simulink model "PC_Quadcopter_Simulation_AE_sslee"  (R2023b)
settings: Solver=ode4  StartTime=0.0  StopTime=40  FixedStep=0.002  MaxStep=0.06  RelTol=1e-3
PreLoadFcn:
  | DoB_parameter
model workspace (MAT data in the model file):
  Sig = Simulink.Signal
  Sig.DataType = 'auto'
  Sig.Dimensions = -1
  Sig.DimensionsMode = 'auto'
  Sig.Complexity = 'auto'
  Sig.SampleTime = -1
  Sig.SamplingMode = 'auto'
values from neighbouring files (symbols this model uses):
  IC = block.DialogPrm(2).Data    [quadcopterDynamicsSFunction.m]
undefined symbols (not defined in the file or in its folder): quadModel
libraries: simulink x14
Description:
  | This is a configurable quadcopter simulation.
  | This Simulink model demonstates position control.
  | 
  | Additional quadcopter modeling and simulation materials available at:
  | github.com/dch33/Quad-Sim
  | 
  | Copyright (C) 2014 D. Hartman, K. Landis, S. Moreno, J. Kim, M. Mehrer
  | 
  | License:
  |     This program is free software: you can redistribute it and/or modify
  |     it under the terms of the GNU LESSER GENERAL PUBLIC LICENSE as published by
  |     the Free Software Foundation, either version 3 of the License, or
  |     (at your option) any later version.
  | 
  |     This program is distributed in the hope that it will be useful,
  |     but WITHOUT ANY WARRANTY; without even the implied warranty of
  |     MERCHANTABILITY or FITNESS FOR A PARTICULAR PURPOSE.  See the
  |     GNU General Public License for more details.
  | 
  |     You should have received a copy of the GNU LESSER GENERAL PUBLIC LICENSE
  |     along with this program.  If not, see <http://www.gnu.org/licenses/>.
settings Model: ModifiedComment=skim -- Tue May 01 16:43:25 2018 -- Version 1.6  Creator=David Hartman  LastModifiedBy=UASG
settings Model: ModifiedHistory=|
  | skim -- Tue May 01 16:43:25 2018 -- Version 1.6
  | 
  | 
  | davidhartman -- Fri Jun 06 22:59:54 2014 -- Version 1.5
settings SolverCC: AlgebraicLoopSolver=TrustRegion
settings DataIOCC: SaveFormat=Array  SignalLogging=off  ReturnWorkspaceOutputs=off
settings OptimizationCC: DefaultParameterBehavior=Inlined  LifeSpan=inf
settings DebuggingCC: SolverPrmCheckMsg=warning  UnconnectedInputMsg=warning  UnconnectedOutputMsg=warning  UnconnectedLineMsg=warning  UniqueDataStoreMsg=warning  StateNameClashWarn=warning  StrictBusMsg=ErrorOnBusTreatedAsVector  SFUnexpectedBacktrackingDiag=warning  SFNoUnconditionalDefaultTransitionDiag=warning  SFExecutionAtInitializationDiag=none  ArithmeticOperatorsInVariantConditions=warning
settings HardwareCC: ProdBitPerPointer=32  ProdBitPerSizeT=32  ProdBitPerPtrDiffT=32  ProdLargestAtomicFloat=None  ProdIntDivRoundTo=Undefined  ProdEndianess=Unspecified  ProdWordSize=32  ProdHWDeviceType=32-bit Generic
settings ModelReferenceCC: EnableRefExpFcnMdlSchedulingChecks=on  PropagateSignalLabelsOutOfModel=off
settings SFSimCC: SimUseLocalCustomCode=off  CustomCodeUndefinedFunction=UseInterfaceOnly
settings RTWCC: RTWUseLocalCustomCode=off  DLArmComputeVersion=19.05
settings CodeAppCC: StateflowObjectComments=on
settings GRTTargetCC: TargetLangStandard=C89/C90 (ANSI)
settings ConfigComp: CovMetricSettings=dw  CovSaveCumulativeToWorkspaceVar=on  CovSaveSingleToWorkspaceVar=on  CovExternalEMLEnable=off

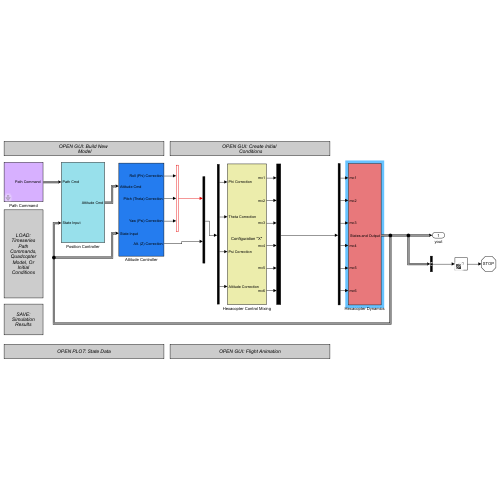
[thumbnail: Simulink's stored preview of the top-level diagram]
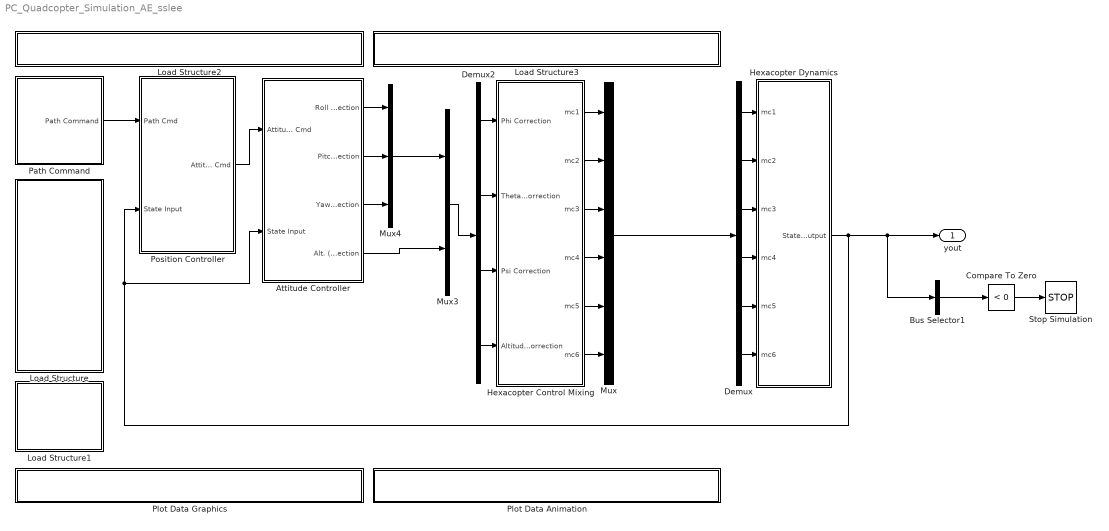
== system PC_Quadcopter_Simulation_AE_sslee ==
  Attitude Controller : Subsystem
  Bus Selector1 : BusSelector  OutputSignals=Z  OutputAsBus=on
  Compare To Zero : simulink/Logic and Bit Operations/Compare To Zero  relop=<  OutDataTypeStr=boolean
  Demux : Demux  Outputs=6
  Demux2 : Demux
  Hexacopter Control Mixing : Subsystem
      mask Display:
      | modelLoaded = evalin('base','exist(''quadModel'',''var'')');
      | if (modelLoaded==1)
      |     if (evalin('base','quadModel.plusConfig'))
      |     fprintf([' \n' ' \n'  'Configuration "+"']);
      |     else if (~evalin('base','quadModel.plusConfig'))
      |         fprintf([' \n' ' \n' 'Configuration "X"']);
      |         end
      |     end
      | else
      |     fprintf([' \n' ' \n'  'Model Not Loaded']);
      | end
  Hexacopter Dynamics : Subsystem
  Load Structure : Subsystem
      settings: OpenFcn=|
      | uiopen('load')
      | if ((exist('IC')==1) && (exist('quadModel')==1) && (exist('path')==1))
      | set_param(bdroot, 'SimulationCommand', 'update')
      | end
      mask Display: fprintf('LOAD:\nTimeseries\nPath\nCommands,\nQuadcopter\nModel, Or\nInitial\nConditions');
  Load Structure1 : Subsystem
      settings: OpenFcn=|
      | if (exist('IC')==1 && exist('quadModel')==1 && exist('yout') && exist('tout'))
      | saveSimResults()
      | else
      | msgbox('No Data To Save!')
      | end
      mask Display: fprintf('SAVE:\nSimulation\nResults');
  Load Structure2 : Subsystem
      settings: OpenFcn=|
      | if exist('GUI_Modeling') == 2,
      | run('GUI_Modeling')
      | 
      | else
      | 
      | msgbox('The desired GUI must be first added to MATLABs path.')
      | 
      | end
      mask Display: fprintf('OPEN GUI: Build New \n Model');
  Load Structure3 : Subsystem
      settings: OpenFcn=|
      | if exist('GUI_IC') == 2,
      | run('GUI_IC')
      | 
      | else
      | 
      | msgbox('The desired GUI must be first added to MATLABs path.')
      | 
      | end
      mask Display: fprintf('OPEN GUI: Create Initial \n Conditions');
  Mux : Mux  Inputs=6
  Mux3 : Mux  Inputs=2
  Mux4 : Mux  Inputs=3
  Path Command : Subsystem  mask{Interpolate=on, OutputAfterFinalValue=Holding final value}
      mask prompts: Interpolate "Interpolate X, Y, Z, and Psi command data?"; OutputAfterFinalValue "Form output after final data value by:"
      mask help:
      | Selecting the Interpolate data checkbox causes position commands to be
      | linearly interpolated. For additional options related to the Timeseries
      | "path" commands, look under the block and click on the Timeseries From
      | Workspace blocks.
      mask TypeOptions Interpolate: X Timeseries From Wkspace/Interpolate | Y Timeseries From Wkspace/Interpolate | Z Timeseries From Wkspace/Interpolate | Psi Timeseries From Wkspace/Interpolate
      mask TypeOptions OutputAfterFinalValue: X Timeseries From Wkspace/OutputAfterFinalValue | Y Timeseries From Wkspace/OutputAfterFinalValue | Z Timeseries From Wkspace/OutputAfterFinalValue | Psi Timeseries From Wkspace/OutputAfterFinalValue
  Plot Data Animation : Subsystem
      settings: OpenFcn=|
      | if exist('QuadAnim4') == 2,
      |     if exist('yout')
      | 	run('QuadAnim4');
      |     else
      |     msgbox('Simulation must be run before data can be plotted.');
      |     end
      | else                                                                          msgbox('The desired GUI must be first added to MATLABs path.')
      | end
      mask Display: fprintf('OPEN GUI: Flight Animation')
  Plot Data Graphics : Subsystem
      settings: OpenFcn=|
      | if exist('yout')
      | yout = evalin('base', 'yout');
      | tout = evalin('base', 'tout');
      | quadPlots(yout, tout)
      | else
      | msgbox('Simulation must be run before data can be plotted.')
      | end
      mask Display: fprintf('OPEN PLOT: State Data')
  Position Controller : Subsystem
  Stop Simulation : Stop
  yout : Outport
  wires:
  Hexacopter Dynamics/1(States and Output) -> Bus Selector1/1, yout/1, Position Controller/2(State Input), Attitude Controller/2(State Input)
  Path Command/1("Path Command ") -> Position Controller/1(Path Cmd)
  Position Controller/1(Attitude Cmd) -> Attitude Controller/1(Attitude Cmd)
  Mux/1 -> Demux/1
  Hexacopter Control Mixing/2(mc2) -> Mux/2
  Hexacopter Control Mixing/3(mc3) -> Mux/3
  Hexacopter Control Mixing/1(mc1) -> Mux/1
  Hexacopter Control Mixing/4(mc4) -> Mux/4
  Demux/3 -> Hexacopter Dynamics/3(mc3)
  Demux/4 -> Hexacopter Dynamics/4(mc4)
  Demux/1 -> Hexacopter Dynamics/1(mc1)
  Demux/2 -> Hexacopter Dynamics/2(mc2)
  Attitude Controller/3(Yaw (Psi) Correction) -> Mux4/3
  Attitude Controller/1(Roll (Phi) Correction) -> Mux4/1
  Attitude Controller/2(Pitch (Theta) Correction) -> Mux4/2
  Demux2/3 -> Hexacopter Control Mixing/3(Psi Correction)
  Demux2/4 -> Hexacopter Control Mixing/4(Altitude Correction)
  Demux2/2 -> Hexacopter Control Mixing/2(Theta Correction)
  Demux2/1 -> Hexacopter Control Mixing/1(Phi Correction)
  Mux4/1 -> Mux3/1
  Attitude Controller/4(Alt. (Z) Correction) -> Mux3/2
  Mux3/1 -> Demux2/1
  Hexacopter Control Mixing/5(mc5) -> Mux/5
  Hexacopter Control Mixing/6(mc6) -> Mux/6
  Demux/5 -> Hexacopter Dynamics/5(mc5)
  Demux/6 -> Hexacopter Dynamics/6(mc6)
  Bus Selector1/1 -> Compare To Zero/1
  Compare To Zero/1 -> Stop Simulation/1

== system PC_Quadcopter_Simulation_AE_sslee/Attitude Controller ==
  Attitude Cmd : Inport
  State Input : Inport  Port=2
  Altitude (Z) Control : Subsystem  mask{Kpz=9, Kiz=6.6, Kdz=9.9, LimitOutput=on, USat=1, LSat=-1, GOffset=(sqrt((quadModel.mass*quadModel.g)/(6*quadModel.ct))-quadModel.b)/quadModel.cr}
      mask prompts: Kpz "Kp"; Kiz "Ki"; Kdz "Kd"; LimitOutput "Integral Saturation?"; USat "Upper saturation limit:"; LSat "Lower saturation limit:"; GOffset "Gravity Feedforward"
      mask help:
      | Adjust PID controller gains through this mask interface, or "look under mask" for more detailed adjustments.
      |
      | Note: Gravity Offset will not appear on block face as a value until simulation is run if it is the result of a formula involving the quadcopter model parameters.
      mask TypeOptions Kpz: Kpz/Gain
      mask TypeOptions Kiz: Kiz/Gain
      mask TypeOptions Kdz: Kdz/Gain
      mask TypeOptions LimitOutput:
      | Integrator
      | Limited/LimitOutput
      mask TypeOptions USat:
      | Integrator
      | Limited/UpperSaturationLimit
      mask TypeOptions LSat:
      | Integrator
      | Limited/LowerSaturationLimit
      mask TypeOptions GOffset: Gravity Offset (Level Flight)/Value
      mask Display:
      | fprintf(['Gravity Offset = ' num2str(GOffset) '\n' ...
      |     'Kp = ' num2str(Kpz) '\n' ...
      |     'Ki = ' num2str(Kiz) '\n' ...
      |     'Kd = ' num2str(Kdz) '\n' ...
      |     'Integral Saturation: ' LimitOutput]);
      | if strcmp(LimitOutput,'on')
      |     fprintf([' \n' ' \n' ' \n' ' \n' ' \n' '\n' ...
      |         'Limits: ' num2str(USat) ' to ' num2str(LSat)]);
      | end
  Bus Selector : BusSelector  OutputSignals=Phi,P,The,Q,Psi,R,Z
  Pitch (Theta) Control : Subsystem  mask{Kpt=2, Kit=1.1, Kdt=1.2, LimitOutput=on, USat=1, LSat=-1}
      mask prompts: Kpt "Kp"; Kit "Ki"; Kdt "Kd"; LimitOutput "Integral Saturation?"; USat "Upper saturation limit:"; LSat "Lower saturation limit:"
      mask help: Adjust PID controller gains through this mask interface, or "look under mask" for more detailed adjustments.
      mask TypeOptions Kpt: Kpt/Gain
      mask TypeOptions Kit: Kit/Gain
      mask TypeOptions Kdt: Kdt/Gain
      mask TypeOptions LimitOutput:
      | Integrator
      | Limited/LimitOutput
      mask TypeOptions USat:
      | Integrator
      | Limited/UpperSaturationLimit
      mask TypeOptions LSat:
      | Integrator
      | Limited/LowerSaturationLimit
      mask Display:
      | fprintf(['Kp = ' num2str(Kpt) '\n' ...
      |     'Ki = ' num2str(Kit) '\n' ...
      |     'Kd = ' num2str(Kdt) '\n' ...
      |     'Integral Saturation: ' LimitOutput]);
      | if strcmp(LimitOutput,'on')
      |     fprintf([' \n' ' \n' ' \n' ' \n' '\n' ...
      |         'Limits: ' num2str(USat) ' to ' num2str(LSat)]);
      | end
  "Roll (Phi) Control " : Subsystem  mask{Kpp=2, Kip=1.1, Kdp=1.2, LimitOutput=on, USat=1, LSat=-1}
      mask prompts: Kpp "Kp"; Kip "Ki"; Kdp "Kd"; LimitOutput "Integral Saturation:"; USat "Upper saturation limit:"; LSat "Lower saturation limit:"
      mask help:
      | Adjust PID controller gains through this mask interface, or "look under mask"
      | for more detailed adjustments.
      mask TypeOptions Kpp: Kpp/Gain
      mask TypeOptions Kip: Kip/Gain
      mask TypeOptions Kdp: Kdp/Gain
      mask TypeOptions LimitOutput:
      | Integrator
      | Limited/LimitOutput
      mask TypeOptions USat:
      | Integrator
      | Limited/UpperSaturationLimit
      mask TypeOptions LSat:
      | Integrator
      | Limited/LowerSaturationLimit
      mask Display:
      | fprintf(['Kp = ' num2str(Kpp) '\n' ...
      |     'Ki = ' num2str(Kip) '\n' ...
      |     'Kd = ' num2str(Kdp) '\n'...
      |     'Integral Saturation: ' LimitOutput]);
      | if strcmp(LimitOutput,'on')
      |     fprintf([' \n' ' \n' ' \n' ' \n' '\n' ...
      |         'Limits: ' num2str(USat) ' to ' num2str(LSat)]);
      | end
  Yaw (Psi) Control : Subsystem  mask{Kps=0.3, Kis=0.15, Kds=0.5, LimitOutput=on, USat=1, LSat=-1}
      mask prompts: Kps "Kp"; Kis "Ki"; Kds "Kd"; LimitOutput "Integral Saturation?"; USat "Upper saturation limit:"; LSat "Lower saturation limit:"
      mask help: Adjust PID controller gains through this mask interface, or "look under mask" for more detailed adjustments.
      mask TypeOptions Kps: Kps/Gain
      mask TypeOptions Kis: Kit/Gain
      mask TypeOptions Kds: Kds/Gain
      mask TypeOptions LimitOutput:
      | Integrator
      | Limited/LimitOutput
      mask TypeOptions USat:
      | Integrator
      | Limited/UpperSaturationLimit
      mask TypeOptions LSat:
      | Integrator
      | Limited/LowerSaturationLimit
      mask Display:
      | fprintf(['Kp = ' num2str(Kps) '\n' ...
      |     'Ki = ' num2str(Kis) '\n' ...
      |     'Kd = ' num2str(Kds) '\n' ...
      |     'Integral Saturation: ' LimitOutput]);
      | if strcmp(LimitOutput,'on')
      |     fprintf([' \n' ' \n' ' \n' ' \n' '\n' ...
      |         'Limits: ' num2str(USat) ' to ' num2str(LSat)]);
      | end
  Roll (Phi) Correction : Outport
  Pitch (Theta) Correction : Outport  Port=2
  Yaw (Psi) Correction : Outport  Port=3
  Alt. (Z) Correction : Outport  Port=4
  wires:
  "Roll (Phi) Control "/1(Phi Correction) -> Roll (Phi) Correction/1
  Bus Selector/1 -> "Roll (Phi) Control "/2(Phi State)  "<Phi>"
  State Input/1 -> Bus Selector/1
  Pitch (Theta) Control/1(Theta Correction) -> Pitch (Theta) Correction/1
  Yaw (Psi) Control/1(Psi Correction) -> Yaw (Psi) Correction/1
  Bus Selector/5 -> Yaw (Psi) Control/2(Psi State)  "<Psi>"
  Altitude (Z) Control/1(Alt. (Z) Correction) -> Alt. (Z) Correction/1
  Bus Selector/7 -> Altitude (Z) Control/2(Z State)  "<Z>"
  Attitude Cmd/1 -> Altitude (Z) Control/1(Desired Z), Yaw (Psi) Control/1(Attitude Command), Pitch (Theta) Control/1(Attitude Command), "Roll (Phi) Control "/1("Attitude Command ")
  Bus Selector/3 -> Pitch (Theta) Control/2(Theta State)  "<The>"
  Bus Selector/2 -> "Roll (Phi) Control "/3(P)  "<P>"
  Bus Selector/4 -> Pitch (Theta) Control/3(P State)  "<Q>"
  Bus Selector/6 -> Yaw (Psi) Control/3(R State)  "<R>"

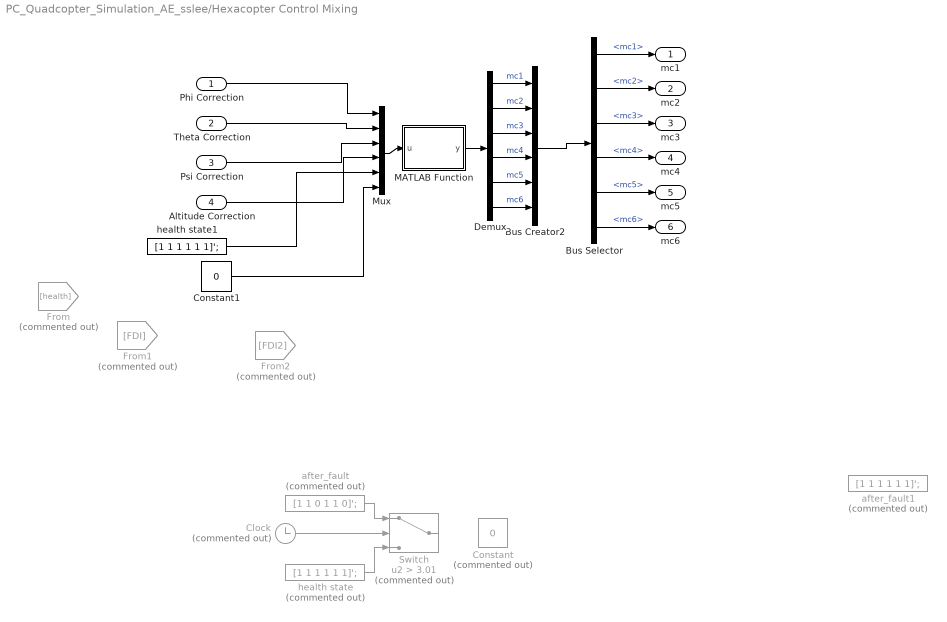
== system PC_Quadcopter_Simulation_AE_sslee/Hexacopter Control Mixing ==
  Phi Correction : Inport
  Theta Correction : Inport  Port=2
  Psi Correction : Inport  Port=3
  Altitude Correction : Inport  Port=4
  Bus Creator2 : BusCreator  Inputs=6
  Bus Selector : BusSelector  OutputSignals=mc1,mc2,mc3,mc4,mc5,mc6
  Clock : Clock  Commented=on
  Constant : Constant  Commented=on  Value=0
  Constant1 : Constant  Value=0
  Demux : Demux  Outputs=6
  From : From  Commented=on  GotoTag=health  TagVisibility=global
  From1 : From  Commented=on  GotoTag=FDI  TagVisibility=global
  From2 : From  Commented=on  GotoTag=FDI2  TagVisibility=global
  MATLAB Function : MATLAB Function  TreatAsAtomicUnit=on
  Mux : Mux  Inputs=6
  Switch : Switch  Commented=on  Criteria=u2 > Threshold  Threshold=3.01  SaturateOnIntegerOverflow=off  InputSameDT=off
  after_fault : Constant  Commented=on  Value=[1 1 0 1 1 0]';
  after_fault1 : Constant  Commented=on  Value=[1 1 1 1 1 1]';
  health state : Constant  Commented=on  Value=[1 1 1 1 1 1]';
  health state1 : Constant  Value=[1 1 1 1 1 1]';
  mc1 : Outport
  mc2 : Outport  Port=2
  mc3 : Outport  Port=3
  mc4 : Outport  Port=4
  mc5 : Outport  Port=5
  mc6 : Outport  Port=6
  wires:
  Phi Correction/1 -> Mux/1
  Theta Correction/1 -> Mux/2
  Psi Correction/1 -> Mux/3
  Altitude Correction/1 -> Mux/4
  Bus Selector/1 -> mc1/1  "<mc1>"
  Bus Selector/2 -> mc2/1  "<mc2>"
  Bus Selector/3 -> mc3/1  "<mc3>"
  Bus Selector/4 -> mc4/1  "<mc4>"
  Bus Selector/5 -> mc5/1  "<mc5>"
  Bus Selector/6 -> mc6/1  "<mc6>"
  Mux/1 -> MATLAB Function/1(u)
  MATLAB Function/1(y) -> Demux/1
  Demux/6 -> Bus Creator2/6  "mc6"
  Demux/3 -> Bus Creator2/3  "mc3"
  Demux/4 -> Bus Creator2/4  "mc4"
  Demux/1 -> Bus Creator2/1  "mc1"
  Demux/5 -> Bus Creator2/5  "mc5"
  Demux/2 -> Bus Creator2/2  "mc2"
  Bus Creator2/1 -> Bus Selector/1
  Constant1/1 -> Mux/6
  health state1/1 -> Mux/5
  health state/1 -> Switch/3
  after_fault/1 -> Switch/1
  Clock/1 -> Switch/2

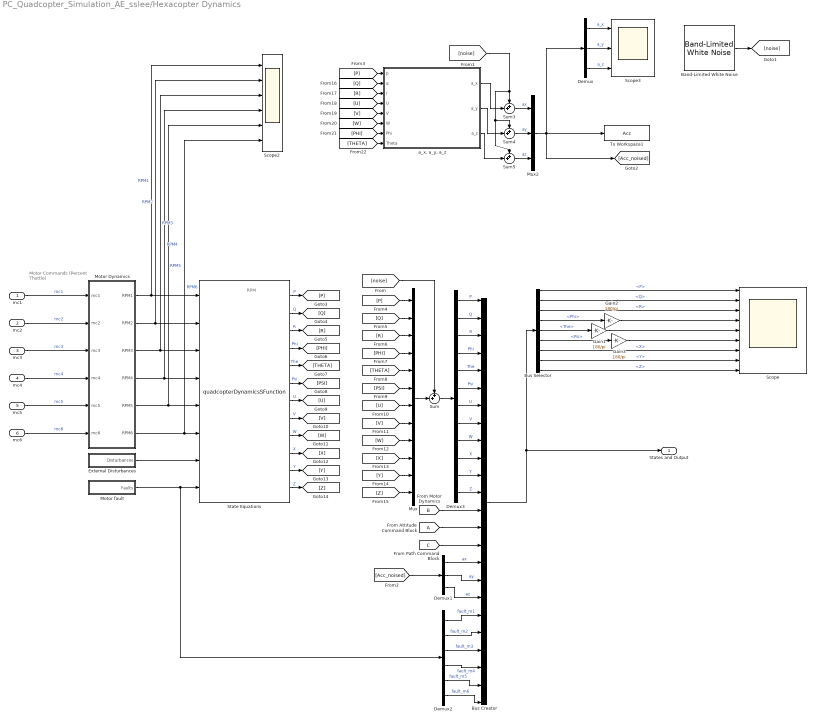
== system PC_Quadcopter_Simulation_AE_sslee/Hexacopter Dynamics ==
  note: RPM
  note: Motor Commands
      | (Percent Thottle)
  mc1 : Inport
  mc2 : Inport  Port=2
  mc3 : Inport  Port=3
  mc4 : Inport  Port=4
  mc5 : Inport  Port=5
  mc6 : Inport  Port=6
  Band-Limited White Noise : simulink/Sources/Band-Limited White Noise  Cov=1e-6  Ts=0.01  seed=[23341]
  Bus Creator : BusCreator  Inputs=24
  Bus Selector : BusSelector  OutputSignals=P,Q,R,Phi,The,Psi,X,Y,Z
  Demux : Demux  Outputs=3
  Demux1 : Demux  Outputs=3
  Demux2 : Demux  Outputs=6
  Demux3 : Demux  Outputs=12
  External Disturbances : Subsystem
  From Attitude Command Block : From  TagVisibility=global
  Gain1 : Gain  Gain=180/pi
  Gain2 : Gain  Gain=180/pi
  Gain3 : Gain  Gain=180/pi
  Motor Dynamics : Subsystem
  Motor fault : Subsystem
  Mux : Mux  Inputs=12
  Mux2 : Mux  Inputs=3
  Scope : Scope  NumInputPorts=9
  Scope2 : Scope  NumInputPorts=6
  Scope3 : Scope  NumInputPorts=3
  State Equations : M-S-Function  FunctionName=quadcopterDynamicsSFunction  Parameters=quadModel, IC
      mask Display:
      | port_label('input', 1, 'RPM1')
      | port_label('input', 2, 'RPM2')
      | port_label('input', 3, 'RPM3')
      | port_label('input', 4, 'RPM4')
      | port_label('input', 5, 'RPM5')
      | port_label('input', 6, 'RPM6')
      | port_label('input', 7, 'Disturbances')
      | port_label('input', 8, 'Faults')
      | port_label('output', 1, 'P')
      | port_label('output', 2, 'Q')
      | port_label('output', 3, 'R')
      | port_label('output', 4, 'Phi')
      | port_label('output', 5, 'The')
      | port_label('output', 6, 'Psi')
      | port_label('output', 7, 'U')
      | port_label('output', 8, 'V')
      | port_label('output', 9, 'W')
      | port_label('output', 10, 'X')
      | port_label('output', 11, 'Y')
      | port_label('output', 12, 'Z')
  Sum{,3..5} (4 alike) : Sum  Inputs=++|
  To Workspace1 : ToWorkspace  VariableName=Acc  SaveFormat=Structure  SampleTime=-1
      settings: Save2DSignal=2-D array (concatenate along first dimension)
  "a_x, a_y, a_z" : Subsystem
  States and Output : Outport
  wires:
  Bus Creator/1 -> Bus Selector/1, States and Output/1
  Motor Dynamics/1(RPM1) -> Scope2/1, State Equations/1  "RPM1"
  Motor Dynamics/2(RPM2) -> Scope2/2, State Equations/2  "RPM2"
  Motor Dynamics/3(RPM3) -> Scope2/3, State Equations/3  "RPM3"
  Motor Dynamics/4(RPM4) -> State Equations/4, Scope2/4  "RPM4"
  mc1/1 -> Motor Dynamics/1(mc1)  "mc1"
  mc4/1 -> Motor Dynamics/4(mc4)  "mc4"
  mc3/1 -> Motor Dynamics/3(mc3)  "mc3"
  mc2/1 -> Motor Dynamics/2(mc2)  "mc2"
  External Disturbances/1("Disturbances ") -> State Equations/7
  From Attitude Command Block/1 -> Bus Creator/14
  [B] -> Bus Creator/13
  [C] -> Bus Creator/15
  mc5/1 -> Motor Dynamics/5(mc5)  "mc5"
  mc6/1 -> Motor Dynamics/6(mc6)  "mc6"
  Motor Dynamics/5(RPM5) -> State Equations/5, Scope2/5  "RPM5"
  Motor Dynamics/6(RPM6) -> State Equations/6, Scope2/6  "RPM6"
  Motor fault/1(Faults) -> Demux2/1, State Equations/8
  Bus Selector/1 -> Scope/1  "<P>"
  Bus Selector/2 -> Scope/2  "<Q>"
  Bus Selector/3 -> Scope/3  "<R>"
  Bus Selector/4 -> Gain2/1  "<Phi>"
  Bus Selector/5 -> Gain1/1  "<The>"
  Bus Selector/6 -> Gain3/1  "<Psi>"
  Bus Selector/7 -> Scope/7  "<X>"
  Bus Selector/8 -> Scope/8  "<Y>"
  Bus Selector/9 -> Scope/9  "<Z>"
  Gain1/1 -> Scope/5
  Gain2/1 -> Scope/4
  Gain3/1 -> Scope/6
  Demux/3 -> Scope3/3  "a_z"
  Demux/2 -> Scope3/2  "a_y"
  Demux/1 -> Scope3/1  "a_x"
  Mux2/1 -> [Acc_noised], To Workspace1/1, Demux/1
  Band-Limited White Noise/1 -> [noise]
  "a_x, a_y, a_z"/1(a_x) -> Sum3/2
  Sum3/1 -> Mux2/1  "ax"
  "a_x, a_y, a_z"/2(a_y) -> Sum4/2
  Sum4/1 -> Mux2/2  "ay"
  "a_x, a_y, a_z"/3(a_z) -> Sum5/2
  Sum5/1 -> Mux2/3  "az"
  [noise] -> Sum5/1, Sum4/1, Sum3/1
  [Acc_noised] -> Demux1/1
  Demux1/1 -> Bus Creator/16  "ax"
  Demux1/2 -> Bus Creator/17  "ay"
  Demux1/3 -> Bus Creator/18  "az"
  Demux2/1 -> Bus Creator/19  "fault_m1"
  Demux2/2 -> Bus Creator/20  "fault_m2"
  Demux2/4 -> Bus Creator/22  "fault_m4"
  Demux2/3 -> Bus Creator/21  "fault_m3"
  Demux2/5 -> Bus Creator/23  "fault_m5"
  Demux2/6 -> Bus Creator/24  "fault_m6"
  State Equations/1 -> [P]  "P"
  State Equations/2 -> [Q]  "Q"
  State Equations/3 -> [R]  "R"
  State Equations/4 -> [PHI]  "Phi"
  State Equations/5 -> [THETA]  "The"
  State Equations/6 -> [PSI]  "Psi"
  State Equations/7 -> [U]  "U"
  State Equations/8 -> [V]  "V"
  State Equations/9 -> [W]  "W"
  State Equations/10 -> [X]  "X"
  State Equations/11 -> [Y]  "Y"
  State Equations/12 -> [Z]  "Z"
  [P] -> "a_x, a_y, a_z"/1(p)
  [Q] -> "a_x, a_y, a_z"/2(q)
  [R] -> "a_x, a_y, a_z"/3(r)
  [U] -> "a_x, a_y, a_z"/4(U)
  [V] -> "a_x, a_y, a_z"/5(V)
  [W] -> "a_x, a_y, a_z"/6(W)
  [THETA] -> "a_x, a_y, a_z"/8(Theta)
  [PHI] -> "a_x, a_y, a_z"/7(Phi)
  [P] -> Mux/1
  [Q] -> Mux/2
  [R] -> Mux/3
  Demux3/1 -> Bus Creator/1  "P"
  Demux3/2 -> Bus Creator/2  "Q"
  Demux3/3 -> Bus Creator/3  "R"
  Mux/1 -> Sum/2
  Sum/1 -> Demux3/1
  [noise] -> Sum/1
  [PHI] -> Mux/4
  [THETA] -> Mux/5
  [PSI] -> Mux/6
  [U] -> Mux/7
  [V] -> Mux/8
  [W] -> Mux/9
  [X] -> Mux/10
  [Y] -> Mux/11
  [Z] -> Mux/12
  Demux3/4 -> Bus Creator/4  "Phi"
  Demux3/5 -> Bus Creator/5  "The"
  Demux3/6 -> Bus Creator/6  "Psi"
  Demux3/7 -> Bus Creator/7  "U"
  Demux3/8 -> Bus Creator/8  "V"
  Demux3/9 -> Bus Creator/9  "W"
  Demux3/10 -> Bus Creator/10  "X"
  Demux3/11 -> Bus Creator/11  "Y"
  Demux3/12 -> Bus Creator/12  "Z"

== system PC_Quadcopter_Simulation_AE_sslee/Load Structure ==

== system PC_Quadcopter_Simulation_AE_sslee/Load Structure1 ==

== system PC_Quadcopter_Simulation_AE_sslee/Load Structure2 ==

== system PC_Quadcopter_Simulation_AE_sslee/Load Structure3 ==

== system PC_Quadcopter_Simulation_AE_sslee/Path Command ==
  Bus Creator : BusCreator  Inputs=4
  Bus Selector : BusSelector  OutputSignals=X_cmd,Y_cmd  OutputAsBus=on
  Psi Timeseries From Wkspace : FromWorkspace  VariableName=path.psi  OutputAfterFinalValue=Holding final value
  X Timeseries From Wkspace : FromWorkspace  VariableName=path.x  OutputAfterFinalValue=Holding final value
  Y Timeseries From Wkspace : FromWorkspace  VariableName=path.y  OutputAfterFinalValue=Holding final value
  Z Timeseries From Wkspace : FromWorkspace  VariableName=path.z  OutputAfterFinalValue=Holding final value
  "Path Command " : Outport
  tag scope: C=global
  wires:
  X Timeseries From Wkspace/1 -> Bus Creator/1  "X_cmd"
  Y Timeseries From Wkspace/1 -> Bus Creator/2  "Y_cmd"
  Z Timeseries From Wkspace/1 -> Bus Creator/3  "Alt_Cmd"
  Psi Timeseries From Wkspace/1 -> Bus Creator/4  "Psi_cmd"
  Bus Creator/1 -> Bus Selector/1, "Path Command "/1  "Path_Cmd"
  Bus Selector/1 -> [C]  "XY_Cmd"

== system PC_Quadcopter_Simulation_AE_sslee/Plot Data Animation ==

== system PC_Quadcopter_Simulation_AE_sslee/Plot Data Graphics ==

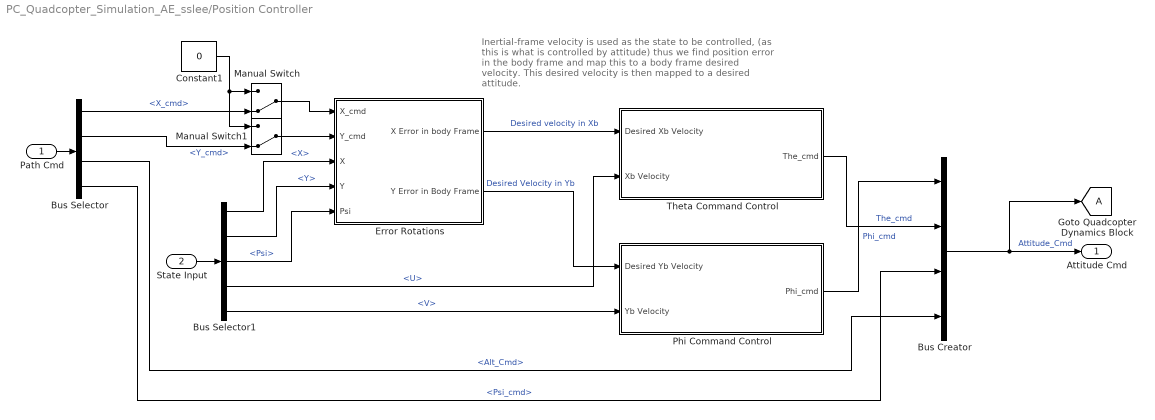
== system PC_Quadcopter_Simulation_AE_sslee/Position Controller ==
  note: Inertial-frame velocity is used as the state to be controlled,
      | (as this is what is controlled by attitude)
      | thus we find position error in the body frame
      | and map this to a body frame desired velocity. This desired
      | velocity is then mapped to a desired attitude.
  Path Cmd : Inport
  State Input : Inport  Port=2
  Bus Creator : BusCreator  Inputs=4
  Bus Selector : BusSelector  OutputSignals=X_cmd,Y_cmd,Alt_Cmd,Psi_cmd
  Bus Selector1 : BusSelector  OutputSignals=X,Y,Psi,U,V
  Constant1 : Constant  Value=0
  Error Rotations : Subsystem
  Goto Quadcopter Dynamics Block : Goto  TagVisibility=global
  Manual Switch : ManualSwitch  CurrentSetting=0
  Manual Switch1 : ManualSwitch  CurrentSetting=0
  Phi Command Control : Subsystem  mask{Kp=0.32, Kd=0.1, ASat=20*pi/180}
      mask prompts: Kp "Proportional Gain"; Kd "Derivative Gain"; ASat "Attitude Limit (+/- radians):"
      mask TypeOptions Kp: Kpp/Gain
      mask TypeOptions Kd: Kdp/Gain
      mask TypeOptions ASat: Attitude Limits_Phi/UpperLimit
      mask Display:
      | fprintf(['Kp = ' num2str(Kp) '\n' ...
      |     'Kd = ' num2str(Kd) '\n' ...
      |     'Attitude Limit (+/-): ' num2str(ASat*180/pi) '°']);
  Theta Command Control : Subsystem  mask{Kp=0.32, Kd=0.1, ASat=20*pi/180}
      mask prompts: Kp "Proportional Gain:"; Kd "Derivative Gain"; ASat "Attitude Limit (+/- radians):"
      mask TypeOptions Kp: Kpt/Gain
      mask TypeOptions Kd: Kdt/Gain
      mask TypeOptions ASat: Attitude Limits_Theta/UpperLimit
      mask Display:
      | fprintf(['Kp = ' num2str(Kp) '\n' ...
      |     'Kd = ' num2str(Kd) '\n' ...
      |     'Attitude Limit (+/-): ' num2str(ASat*180/pi) '°']);
  Attitude Cmd : Outport
  wires:
  Bus Selector1/5 -> Phi Command Control/2(Yb Velocity)  "<V>"
  State Input/1 -> Bus Selector1/1
  Bus Selector/4 -> Bus Creator/3  "<Psi_cmd>"
  Path Cmd/1 -> Bus Selector/1
  Bus Selector/3 -> Bus Creator/4  "<Alt_Cmd>"
  Bus Creator/1 -> Attitude Cmd/1, Goto Quadcopter Dynamics Block/1  "Attitude_Cmd"
  Bus Selector/1 -> Manual Switch/2  "<X_cmd>"
  Bus Selector1/1 -> Error Rotations/3(X)  "<X>"
  Bus Selector1/2 -> Error Rotations/4(Y)  "<Y>"
  Bus Selector1/3 -> Error Rotations/5(Psi)  "<Psi>"
  Error Rotations/1(X Error in body Frame) -> Theta Command Control/1(Desired Xb Velocity)  "Desired velocity in Xb"
  Bus Selector1/4 -> Theta Command Control/2(Xb Velocity)  "<U>"
  Theta Command Control/1(The_cmd) -> Bus Creator/2  "The_cmd"
  Error Rotations/2(Y Error in Body Frame) -> Phi Command Control/1(Desired Yb Velocity)  "Desired Velocity in Yb"
  Phi Command Control/1(Phi_cmd) -> Bus Creator/1  "Phi_cmd"
  Constant1/1 -> Manual Switch1/1, Manual Switch/1
  Manual Switch/1 -> Error Rotations/1(X_cmd)
  Bus Selector/2 -> Manual Switch1/2  "<Y_cmd>"
  Manual Switch1/1 -> Error Rotations/2(Y_cmd)

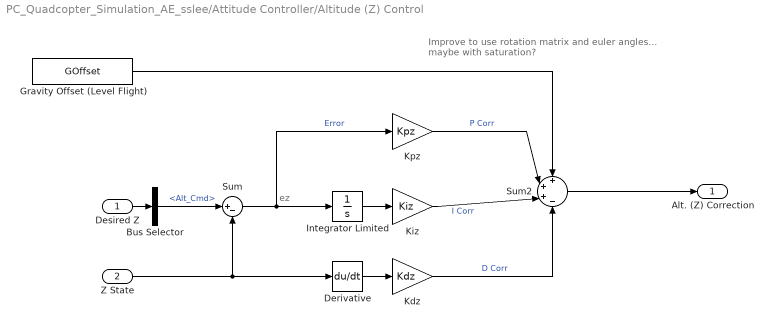
== system PC_Quadcopter_Simulation_AE_sslee/Attitude Controller/Altitude (Z) Control ==
  note: Improve to use rotation matrix and euler angles...
      | maybe with saturation?
  note: ez
  Desired Z : Inport
  Z State : Inport  Port=2
  Bus Selector : BusSelector  OutputSignals=Alt_Cmd
  Derivative : Derivative
  Gravity Offset (Level Flight) : Constant  Value=GOffset
  Integrator Limited : Integrator  LimitOutput=on  UpperSaturationLimit=USat  LowerSaturationLimit=LSat
  Kdz : Gain  Gain=Kdz
  Kiz : Gain  Gain=Kiz
  Kpz : Gain  Gain=Kpz
  Sum : Sum  Inputs=|+-
  Sum2 : Sum  Inputs=+++-
  Alt. (Z) Correction : Outport
  wires:
  Gravity Offset (Level Flight)/1 -> Sum2/1
  Desired Z/1 -> Bus Selector/1
  Z State/1 -> Derivative/1, Sum/2
  Sum2/1 -> Alt. (Z) Correction/1
  Kpz/1 -> Sum2/2  "P Corr"
  Sum/1 -> Integrator Limited/1, Kpz/1  "Error"
  Kiz/1 -> Sum2/3  "I Corr"
  Kdz/1 -> Sum2/4  "D Corr"
  Integrator Limited/1 -> Kiz/1
  Bus Selector/1 -> Sum/1  "<Alt_Cmd>"
  Derivative/1 -> Kdz/1

== system PC_Quadcopter_Simulation_AE_sslee/Attitude Controller/Pitch (Theta) Control ==
  Attitude Command : Inport
  Theta State : Inport  Port=2
  P State : Inport  Port=3
  Bus Selector : BusSelector  OutputSignals=The_cmd
  Integrator Limited : Integrator  LimitOutput=on  UpperSaturationLimit=USat  LowerSaturationLimit=LSat
  Kdt : Gain  Gain=Kdt
  Kit : Gain  Gain=Kit
  Kpt : Gain  Gain=Kpt
  Sum : Sum  Inputs=|+-
  Sum1 : Sum  Inputs=++-
  Theta Correction : Outport
  wires:
  Sum/1 -> Integrator Limited/1, Kpt/1  "Error"
  Attitude Command/1 -> Bus Selector/1
  Theta State/1 -> Sum/2
  Sum1/1 -> Theta Correction/1
  Kpt/1 -> Sum1/1  "P Corr"
  Kdt/1 -> Sum1/3  "D Corr"
  Kit/1 -> Sum1/2  "I Corr"
  Integrator Limited/1 -> Kit/1
  Bus Selector/1 -> Sum/1  "<The_cmd>"
  P State/1 -> Kdt/1

== system PC_Quadcopter_Simulation_AE_sslee/Attitude Controller/Roll (Phi) Control  ==
  "Attitude Command " : Inport
  Phi State : Inport  Port=2
  P : Inport  Port=3
  Bus Selector : BusSelector  OutputSignals=Phi_cmd
  Integrator Limited : Integrator  LimitOutput=on  UpperSaturationLimit=USat  LowerSaturationLimit=LSat
  Kdp : Gain  Gain=Kdp
  Kip : Gain  Gain=Kip
  Kpp : Gain  Gain=Kpp
  Sum : Sum  Inputs=|+-
  Sum1 : Sum  Inputs=++-
  Phi Correction : Outport
  wires:
  Sum/1 -> Integrator Limited/1, Kpp/1  "Error"
  Phi State/1 -> Sum/2
  Sum1/1 -> Phi Correction/1
  Kpp/1 -> Sum1/1  "P Corr"
  Kdp/1 -> Sum1/3  "D Corr"
  Kip/1 -> Sum1/2  "I Corr"
  Integrator Limited/1 -> Kip/1
  "Attitude Command "/1 -> Bus Selector/1
  Bus Selector/1 -> Sum/1  "<Phi_cmd>"
  P/1 -> Kdp/1

== system PC_Quadcopter_Simulation_AE_sslee/Attitude Controller/Yaw (Psi) Control ==
  Attitude Command : Inport
  Psi State : Inport  Port=2
  R State : Inport  Port=3
  Bus Selector : BusSelector  OutputSignals=Psi_cmd
  Integrator Limited : Integrator  LimitOutput=on  UpperSaturationLimit=USat  LowerSaturationLimit=LSat
  Kds : Gain  Gain=Kds
  Kit : Gain  Gain=Kis
  Kps : Gain  Gain=Kps
  Sum : Sum  Inputs=|+-
  Sum1 : Sum  Inputs=++-
  Psi Correction : Outport
  wires:
  Sum/1 -> Integrator Limited/1, Kps/1  "Error"
  Attitude Command/1 -> Bus Selector/1
  Sum1/1 -> Psi Correction/1
  Psi State/1 -> Sum/2
  Kps/1 -> Sum1/1  "P Corr"
  Kds/1 -> Sum1/3  "D Corr"
  Kit/1 -> Sum1/2  "I Corr"
  Integrator Limited/1 -> Kit/1
  Bus Selector/1 -> Sum/1  "<Psi_cmd>"
  R State/1 -> Kds/1

== system PC_Quadcopter_Simulation_AE_sslee/Hexacopter Dynamics/External Disturbances ==
  note: Note: Torques are in units of N*m, Forces in N
      | Torques are applied to the BODY coordinate system.
      | Forces are applied from the WORLD coordinate system!
      | This can be changed by adjusting the equations within the S-function.
  Bus Creator : BusCreator  Inputs=6
  Bus to Vector : BusToVector
  Constant{1..2,5..6} (4 alike) : Constant  Value=0
  Manual Switch : ManualSwitch
  Manual Switch1 : ManualSwitch
  Step : Step  Time=5  After=0.1  SampleTime=0
  Step2 : Step  Time=10  After=3  SampleTime=0
  "Disturbances " : Outport
  wires:
  Bus to Vector/1 -> "Disturbances "/1
  Bus Creator/1 -> Bus to Vector/1
  Constant6/1 -> Manual Switch1/1, Bus Creator/1  "Tau_bx-axis"
  Constant2/1 -> Bus Creator/3  "Tau_bz-axis"
  Constant1/1 -> Manual Switch/1, Bus Creator/4  "Force_x-axis"
  Constant5/1 -> Bus Creator/6  "Force_z-axis"
  Manual Switch/1 -> Bus Creator/5
  Step2/1 -> Manual Switch/2  "Force_y-axis"
  Manual Switch1/1 -> Bus Creator/2
  Step/1 -> Manual Switch1/2  "Tau_by-axis"

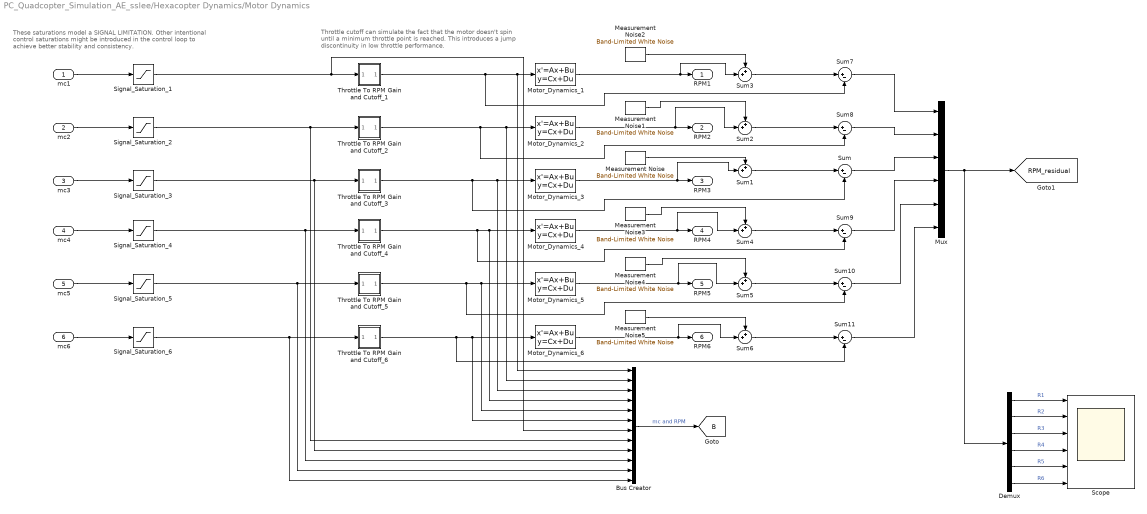
== system PC_Quadcopter_Simulation_AE_sslee/Hexacopter Dynamics/Motor Dynamics ==
  note: Throttle cutoff can simulate the fact that the motor doesn't
      | spin until a minimum throttle point is reached. This introduces
      | a jump discontinuity in low throttle performance.
  note: These saturations model a SIGNAL LIMITATION.
      | Other intentional control saturations might be introduced in the
      | control loop to achieve better stability and consistency.
  mc1 : Inport
  mc2 : Inport  Port=2
  mc3 : Inport  Port=3
  mc4 : Inport  Port=4
  mc5 : Inport  Port=5
  mc6 : Inport  Port=6
  Bus Creator : BusCreator  Inputs=12
  Demux : Demux  Outputs=6
  Measurement Noise{,1..5} (6 alike) : simulink/Sources/Band-Limited White Noise  Cov=10^2  Ts=0.02  seed=[23342]
  Motor_Dynamics_1 : StateSpace  A=-1/quadModel.T  C=1/quadModel.T  D=0  InitialCondition=IC.w1*quadModel.T
  Motor_Dynamics_2 : StateSpace  A=-1/quadModel.T  C=1/quadModel.T  D=0  InitialCondition=IC.w2*quadModel.T
  Motor_Dynamics_3 : StateSpace  A=-1/quadModel.T  C=1/quadModel.T  D=0  InitialCondition=IC.w3*quadModel.T
  Motor_Dynamics_4 : StateSpace  A=-1/quadModel.T  C=1/quadModel.T  D=0  InitialCondition=IC.w4*quadModel.T
  Motor_Dynamics_5 : StateSpace  A=-1/quadModel.T  C=1/quadModel.T  D=0  InitialCondition=IC.w4*quadModel.T
  Motor_Dynamics_6 : StateSpace  A=-1/quadModel.T  C=1/quadModel.T  D=0  InitialCondition=IC.w4*quadModel.T
  Mux : Mux  Inputs=6
  Scope : Scope  NumInputPorts=6
  Signal_Saturation_{1..6} (6 alike) : Saturate  UpperLimit=100  LowerLimit=0
  Sum{,7..11} (6 alike) : Sum  Inputs=|+-
  Sum{1..6} (6 alike) : Sum  Inputs=++|
  Throttle To RPM Gain and Cutoff_1 : Subsystem
  Throttle To RPM Gain and Cutoff_2 : Subsystem
  Throttle To RPM Gain and Cutoff_3 : Subsystem
  Throttle To RPM Gain and Cutoff_4 : Subsystem
  Throttle To RPM Gain and Cutoff_5 : Subsystem
  Throttle To RPM Gain and Cutoff_6 : Subsystem
  RPM1 : Outport
  RPM2 : Outport  Port=2
  RPM3 : Outport  Port=3
  RPM4 : Outport  Port=4
  RPM5 : Outport  Port=5
  RPM6 : Outport  Port=6
  tag scope: B=global, RPM_residual=global
  wires:
  mc1/1 -> Signal_Saturation_1/1
  mc4/1 -> Signal_Saturation_4/1
  mc2/1 -> Signal_Saturation_2/1
  mc3/1 -> Signal_Saturation_3/1
  Signal_Saturation_1/1 -> Bus Creator/7, Throttle To RPM Gain and Cutoff_1/1(In5)
  Signal_Saturation_2/1 -> Throttle To RPM Gain and Cutoff_2/1(In5), Bus Creator/8
  Signal_Saturation_3/1 -> Bus Creator/9, Throttle To RPM Gain and Cutoff_3/1(In5)
  Signal_Saturation_4/1 -> Bus Creator/10, Throttle To RPM Gain and Cutoff_4/1(In5)
  Throttle To RPM Gain and Cutoff_1/1(Out5) -> Sum7/2, Bus Creator/1, Motor_Dynamics_1/1
  Throttle To RPM Gain and Cutoff_2/1(Out5) -> Sum8/2, Motor_Dynamics_2/1, Bus Creator/2
  Throttle To RPM Gain and Cutoff_3/1(Out5) -> Sum/2, Motor_Dynamics_3/1, Bus Creator/3
  Throttle To RPM Gain and Cutoff_4/1(Out5) -> Sum9/2, Motor_Dynamics_4/1, Bus Creator/4
  Motor_Dynamics_1/1 -> Sum3/2, RPM1/1
  Motor_Dynamics_2/1 -> Sum2/2, RPM2/1
  Motor_Dynamics_3/1 -> Sum1/2, RPM3/1
  Motor_Dynamics_4/1 -> Sum4/2, RPM4/1
  Bus Creator/1 -> [B]  "mc and RPM"
  Motor_Dynamics_5/1 -> Sum5/2, RPM5/1
  mc5/1 -> Signal_Saturation_5/1
  Signal_Saturation_5/1 -> Bus Creator/11, Throttle To RPM Gain and Cutoff_5/1(In5)
  Throttle To RPM Gain and Cutoff_5/1(Out5) -> Sum10/2, Motor_Dynamics_5/1, Bus Creator/5
  Motor_Dynamics_6/1 -> Sum6/2, RPM6/1
  mc6/1 -> Signal_Saturation_6/1
  Signal_Saturation_6/1 -> Bus Creator/12, Throttle To RPM Gain and Cutoff_6/1(In5)
  Throttle To RPM Gain and Cutoff_6/1(Out5) -> Sum11/2, Motor_Dynamics_6/1, Bus Creator/6
  Mux/1 -> Demux/1, [RPM_residual]
  Measurement Noise/1 -> Sum1/1
  Sum1/1 -> Sum/1
  Measurement Noise5/1 -> Sum6/1
  Measurement Noise4/1 -> Sum5/1
  Measurement Noise3/1 -> Sum4/1
  Measurement Noise1/1 -> Sum2/1
  Measurement Noise2/1 -> Sum3/1
  Sum2/1 -> Sum8/1
  Sum3/1 -> Sum7/1
  Sum4/1 -> Sum9/1
  Sum5/1 -> Sum10/1
  Sum6/1 -> Sum11/1
  Sum7/1 -> Mux/1
  Sum8/1 -> Mux/2
  Sum/1 -> Mux/3
  Sum9/1 -> Mux/4
  Sum10/1 -> Mux/5
  Sum11/1 -> Mux/6
  Demux/6 -> Scope/6  "R6"
  Demux/5 -> Scope/5  "R5"
  Demux/4 -> Scope/4  "R4"
  Demux/3 -> Scope/3  "R3"
  Demux/2 -> Scope/2  "R2"
  Demux/1 -> Scope/1  "R1"

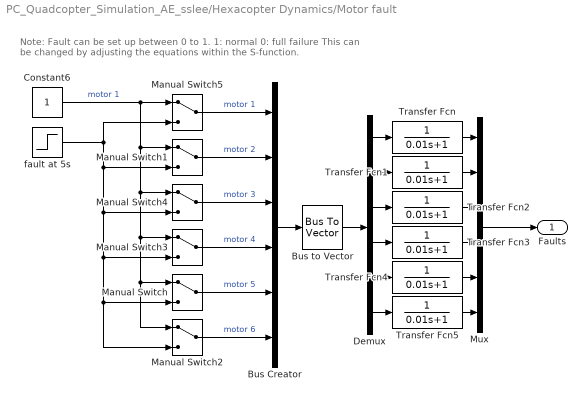
== system PC_Quadcopter_Simulation_AE_sslee/Hexacopter Dynamics/Motor fault ==
  note: Note: Fault can be set up between 0 to 1.
      | 1: normal
      | 0: full failure
      | This can be changed by adjusting the equations within the S-function.
  Bus Creator : BusCreator  Inputs=6
  Bus to Vector : BusToVector
  Constant6 : Constant
  Demux : Demux  Outputs=6
  Manual Switch{,1..5} (6 alike) : ManualSwitch
  Mux : Mux  Inputs=6
  Transfer Fcn{,1..5} (6 alike) : TransferFcn  Numerator=1  Denominator=[0.01 1]
  fault at 5s : Step  Time=30  Before=1  After=0  SampleTime=0
  Faults : Outport
  wires:
  Manual Switch1/1 -> Bus Creator/2  "motor 2"
  Manual Switch/1 -> Bus Creator/5  "motor 5"
  Bus Creator/1 -> Bus to Vector/1
  Manual Switch2/1 -> Bus Creator/6  "motor 6"
  Manual Switch3/1 -> Bus Creator/4  "motor 4"
  Demux/1 -> Transfer Fcn/1
  Demux/2 -> Transfer Fcn1/1
  Demux/3 -> Transfer Fcn2/1
  Demux/6 -> Transfer Fcn5/1
  Demux/5 -> Transfer Fcn4/1
  Demux/4 -> Transfer Fcn3/1
  Transfer Fcn/1 -> Mux/1
  Transfer Fcn1/1 -> Mux/2
  Transfer Fcn2/1 -> Mux/3
  Transfer Fcn4/1 -> Mux/5
  Transfer Fcn5/1 -> Mux/6
  Transfer Fcn3/1 -> Mux/4
  Manual Switch4/1 -> Bus Creator/3  "motor 3"
  Constant6/1 -> Manual Switch5/1, Manual Switch2/1, Manual Switch/1, Manual Switch3/1, Manual Switch4/1, Manual Switch1/1  "motor 1"
  Manual Switch5/1 -> Bus Creator/1  "motor 1"
  fault at 5s/1 -> Manual Switch2/2, Manual Switch/2, Manual Switch3/2, Manual Switch4/2, Manual Switch1/2, Manual Switch5/2
  Bus to Vector/1 -> Demux/1
  Mux/1 -> Faults/1

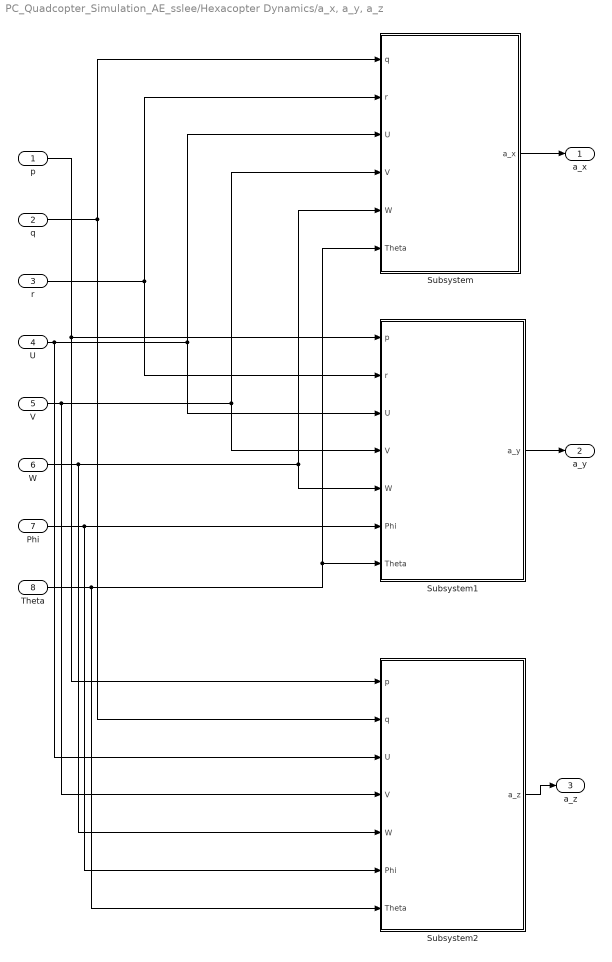
== system PC_Quadcopter_Simulation_AE_sslee/Hexacopter Dynamics/a_x, a_y, a_z ==
  p : Inport
  q : Inport  Port=2
  r : Inport  Port=3
  U : Inport  Port=4
  V : Inport  Port=5
  W : Inport  Port=6
  Phi : Inport  Port=7
  Theta : Inport  Port=8
  Subsystem : Subsystem
  Subsystem1 : Subsystem
  Subsystem2 : Subsystem
  a_x : Outport
  a_y : Outport  Port=2
  a_z : Outport  Port=3
  wires:
  Subsystem/1(a_x) -> a_x/1
  Subsystem1/1(a_y) -> a_y/1
  Subsystem2/1(a_z) -> a_z/1
  q/1 -> Subsystem2/2(q), Subsystem/1(q)
  r/1 -> Subsystem/2(r), Subsystem1/2(r)
  U/1 -> Subsystem2/3(U), Subsystem1/3(U), Subsystem/3(U)
  V/1 -> Subsystem2/4(V), Subsystem/4(V), Subsystem1/4(V)
  W/1 -> Subsystem2/5(W), Subsystem/5(W), Subsystem1/5(W)
  Theta/1 -> Subsystem2/7(Theta), Subsystem1/7(Theta), Subsystem/6(Theta)
  p/1 -> Subsystem2/1(p), Subsystem1/1(p)
  Phi/1 -> Subsystem2/6(Phi), Subsystem1/6(Phi)

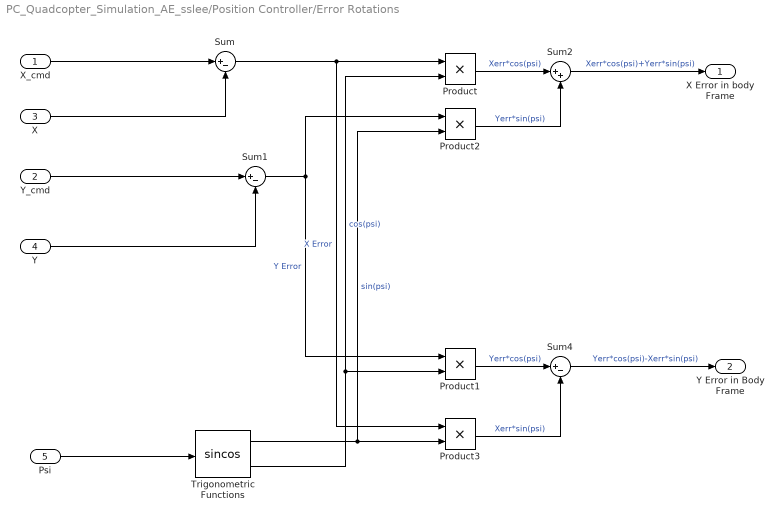
== system PC_Quadcopter_Simulation_AE_sslee/Position Controller/Error Rotations ==
  X_cmd : Inport
  Y_cmd : Inport  Port=2
  X : Inport  Port=3
  Y : Inport  Port=4
  Psi : Inport  Port=5
  Product{,1..3} (4 alike) : Product
  Sum : Sum  Inputs=|+-
  Sum1 : Sum  Inputs=|+-
  Sum2 : Sum  Inputs=|++
  Sum4 : Sum  Inputs=|+-
  Trigonometric Functions : Trigonometry  Operator=sincos
  X Error in body Frame : Outport
  Y Error in Body Frame : Outport  Port=2
  wires:
  Sum4/1 -> Y Error in Body Frame/1  "Yerr*cos(psi)-Xerr*sin(psi)"
  Product3/1 -> Sum4/2  "Xerr*sin(psi)"
  Sum1/1 -> Product2/1, Product1/1  "Y Error"
  Trigonometric Functions/1 -> Product2/2, Product3/2  "sin(psi)"
  Sum2/1 -> X Error in body Frame/1  "Xerr*cos(psi)+Yerr*sin(psi)"
  Y_cmd/1 -> Sum1/1
  X_cmd/1 -> Sum/1
  X/1 -> Sum/2
  Y/1 -> Sum1/2
  Sum/1 -> Product3/1, Product/1  "X Error"
  Trigonometric Functions/2 -> Product/2, Product1/2  "cos(psi)"
  Product/1 -> Sum2/1  "Xerr*cos(psi)"
  Product2/1 -> Sum2/2  "Yerr*sin(psi)"
  Product1/1 -> Sum4/1  "Yerr*cos(psi)"
  Psi/1 -> Trigonometric Functions/1

== system PC_Quadcopter_Simulation_AE_sslee/Position Controller/Phi Command Control ==
  note: -1 Gain is required because a "negative"
      | angle of Phi induces a positive velocity
      | in the body frame y direction!
  Desired Yb Velocity : Inport
  Yb Velocity : Inport  Port=2
  Attitude Limits_Phi : Saturate  UpperLimit=ASat  LowerLimit=-ASat
  Gain : Gain  Gain=-1
  Kdp : Gain  Gain=Kd
  Kpp : Gain  Gain=Kp
  Sum3 : Sum  Inputs=|+-
  Sum6 : Sum  Inputs=|+-
  V Derivative : Derivative
  Phi_cmd : Outport
  wires:
  V Derivative/1 -> Kdp/1
  Attitude Limits_Phi/1 -> Phi_cmd/1  "Phi_cmd"
  Sum6/1 -> Gain/1
  Kpp/1 -> Sum6/1
  Sum3/1 -> Kpp/1  "Velocity Error"
  Yb Velocity/1 -> V Derivative/1, Sum3/2
  Desired Yb Velocity/1 -> Sum3/1
  Gain/1 -> Attitude Limits_Phi/1
  Kdp/1 -> Sum6/2

== system PC_Quadcopter_Simulation_AE_sslee/Position Controller/Theta Command Control ==
  Desired Xb Velocity : Inport
  Xb Velocity : Inport  Port=2
  Attitude Limits_Theta : Saturate  UpperLimit=ASat  LowerLimit=-ASat
  Kdt : Gain  Gain=Kd
  Kpt : Gain  Gain=Kp
  Sum3 : Sum  Inputs=|+-
  Sum6 : Sum  Inputs=|+-
  U Derivative : Derivative
  The_cmd : Outport
  wires:
  Kdt/1 -> Sum6/2
  U Derivative/1 -> Kdt/1
  Attitude Limits_Theta/1 -> The_cmd/1  "The_cmd"
  Sum6/1 -> Attitude Limits_Theta/1
  Kpt/1 -> Sum6/1
  Sum3/1 -> Kpt/1  "Velocity Error"
  Xb Velocity/1 -> U Derivative/1, Sum3/2
  Desired Xb Velocity/1 -> Sum3/1

== system PC_Quadcopter_Simulation_AE_sslee/Hexacopter Dynamics/Motor Dynamics/Throttle To RPM Gain and Cutoff_1 ==
  note: minThr should be a quad.mat value
  note: This gain should be a quad.mat value
  note: This constant should be a quad.mat value
  note: Output equals linearly scaled RPM
      | for given throttle input if throttle input >=Throttle Cuttoff (minThr)
      | else output is zero.
  In5 : Inport
  Constant : Constant  Value=quadModel.b
  Gain : Gain  Gain=quadModel.cr
  Minimum Throttle Cutoff : simulink/Logic and Bit Operations/Compare To Constant  relop=>=  const=quadModel.minThr  OutDataTypeStr=uint8
  Product : Product
  Sum1 : Sum  Inputs=++|
  Out5 : Outport
  wires:
  Minimum Throttle Cutoff/1 -> Product/2
  Product/1 -> Out5/1
  In5/1 -> Gain/1, Minimum Throttle Cutoff/1
  Gain/1 -> Sum1/2
  Sum1/1 -> Product/1
  Constant/1 -> Sum1/1

== system PC_Quadcopter_Simulation_AE_sslee/Hexacopter Dynamics/Motor Dynamics/Throttle To RPM Gain and Cutoff_2 ==
  note: minThr should be a quad.mat value
  note: This gain should be a quad.mat value
  note: This constant should be a quad.mat value
  note: Output equals linearly scaled RPM
      | for given throttle input if throttle input >=Throttle Cuttoff (minThr)
      | else output is zero.
  In5 : Inport
  Constant : Constant  Value=quadModel.b
  Gain : Gain  Gain=quadModel.cr
  Minimum Throttle Cutoff : simulink/Logic and Bit Operations/Compare To Constant  relop=>=  const=quadModel.minThr  OutDataTypeStr=uint8
  Product : Product
  Sum1 : Sum  Inputs=++|
  Out5 : Outport
  wires:
  Minimum Throttle Cutoff/1 -> Product/2
  Product/1 -> Out5/1
  In5/1 -> Gain/1, Minimum Throttle Cutoff/1
  Gain/1 -> Sum1/2
  Sum1/1 -> Product/1
  Constant/1 -> Sum1/1

== system PC_Quadcopter_Simulation_AE_sslee/Hexacopter Dynamics/Motor Dynamics/Throttle To RPM Gain and Cutoff_3 ==
  note: minThr should be a quad.mat value
  note: This gain should be a quad.mat value
  note: This constant should be a quad.mat value
  note: Output equals linearly scaled RPM
      | for given throttle input if throttle input >=Throttle Cuttoff (minThr)
      | else output is zero.
  In5 : Inport
  Constant : Constant  Value=quadModel.b
  Gain : Gain  Gain=quadModel.cr
  Minimum Throttle Cutoff : simulink/Logic and Bit Operations/Compare To Constant  relop=>=  const=quadModel.minThr  OutDataTypeStr=uint8
  Product : Product
  Sum1 : Sum  Inputs=++|
  Out5 : Outport
  wires:
  Minimum Throttle Cutoff/1 -> Product/2
  Product/1 -> Out5/1
  In5/1 -> Gain/1, Minimum Throttle Cutoff/1
  Gain/1 -> Sum1/2
  Sum1/1 -> Product/1
  Constant/1 -> Sum1/1

== system PC_Quadcopter_Simulation_AE_sslee/Hexacopter Dynamics/Motor Dynamics/Throttle To RPM Gain and Cutoff_4 ==
  note: minThr should be a quad.mat value
  note: This gain should be a quad.mat value
  note: This constant should be a quad.mat value
  note: Output equals linearly scaled RPM
      | for given throttle input if throttle input >=Throttle Cuttoff (minThr)
      | else output is zero.
  In5 : Inport
  Constant : Constant  Value=quadModel.b
  Gain : Gain  Gain=quadModel.cr
  Minimum Throttle Cutoff : simulink/Logic and Bit Operations/Compare To Constant  relop=>=  const=quadModel.minThr  OutDataTypeStr=uint8
  Product : Product
  Sum1 : Sum  Inputs=++|
  Out5 : Outport
  wires:
  Minimum Throttle Cutoff/1 -> Product/2
  Product/1 -> Out5/1
  In5/1 -> Gain/1, Minimum Throttle Cutoff/1
  Gain/1 -> Sum1/2
  Sum1/1 -> Product/1
  Constant/1 -> Sum1/1

== system PC_Quadcopter_Simulation_AE_sslee/Hexacopter Dynamics/Motor Dynamics/Throttle To RPM Gain and Cutoff_5 ==
  note: minThr should be a quad.mat value
  note: This gain should be a quad.mat value
  note: This constant should be a quad.mat value
  note: Output equals linearly scaled RPM
      | for given throttle input if throttle input >=Throttle Cuttoff (minThr)
      | else output is zero.
  In5 : Inport
  Constant : Constant  Value=quadModel.b
  Gain : Gain  Gain=quadModel.cr
  Minimum Throttle Cutoff : simulink/Logic and Bit Operations/Compare To Constant  relop=>=  const=quadModel.minThr  OutDataTypeStr=uint8
  Product : Product
  Sum1 : Sum  Inputs=++|
  Out5 : Outport
  wires:
  Minimum Throttle Cutoff/1 -> Product/2
  Product/1 -> Out5/1
  In5/1 -> Gain/1, Minimum Throttle Cutoff/1
  Gain/1 -> Sum1/2
  Sum1/1 -> Product/1
  Constant/1 -> Sum1/1

== system PC_Quadcopter_Simulation_AE_sslee/Hexacopter Dynamics/Motor Dynamics/Throttle To RPM Gain and Cutoff_6 ==
  note: minThr should be a quad.mat value
  note: This gain should be a quad.mat value
  note: This constant should be a quad.mat value
  note: Output equals linearly scaled RPM
      | for given throttle input if throttle input >=Throttle Cuttoff (minThr)
      | else output is zero.
  In5 : Inport
  Constant : Constant  Value=quadModel.b
  Gain : Gain  Gain=quadModel.cr
  Minimum Throttle Cutoff : simulink/Logic and Bit Operations/Compare To Constant  relop=>=  const=quadModel.minThr  OutDataTypeStr=uint8
  Product : Product
  Sum1 : Sum  Inputs=++|
  Out5 : Outport
  wires:
  Minimum Throttle Cutoff/1 -> Product/2
  Product/1 -> Out5/1
  In5/1 -> Gain/1, Minimum Throttle Cutoff/1
  Gain/1 -> Sum1/2
  Sum1/1 -> Product/1
  Constant/1 -> Sum1/1

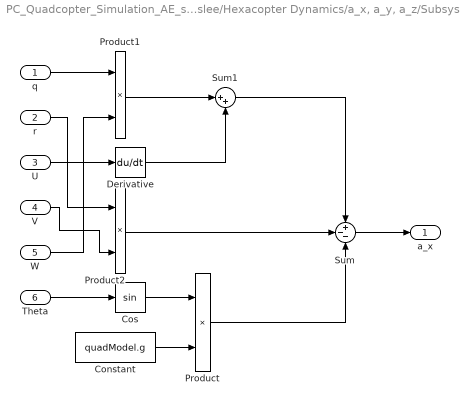
== system PC_Quadcopter_Simulation_AE_sslee/Hexacopter Dynamics/a_x, a_y, a_z/Subsystem ==
  q : Inport
  r : Inport  Port=2
  U : Inport  Port=3
  V : Inport  Port=4
  W : Inport  Port=5
  Theta : Inport  Port=6
  Constant : Constant  Value=quadModel.g
  Cos : Trigonometry
  Derivative : Derivative
  Product : Product
  Product1 : Product
  Product2 : Product
  Sum : Sum  Inputs=+--
  Sum1 : Sum  Inputs=|++
  a_x : Outport
  wires:
  Theta/1 -> Cos/1
  Cos/1 -> Product/1
  Constant/1 -> Product/2
  Product1/1 -> Sum1/1
  Derivative/1 -> Sum1/2
  Sum1/1 -> Sum/1
  Sum/1 -> a_x/1
  Product2/1 -> Sum/2
  Product/1 -> Sum/3
  U/1 -> Derivative/1
  q/1 -> Product1/1
  W/1 -> Product1/2
  r/1 -> Product2/1
  V/1 -> Product2/2

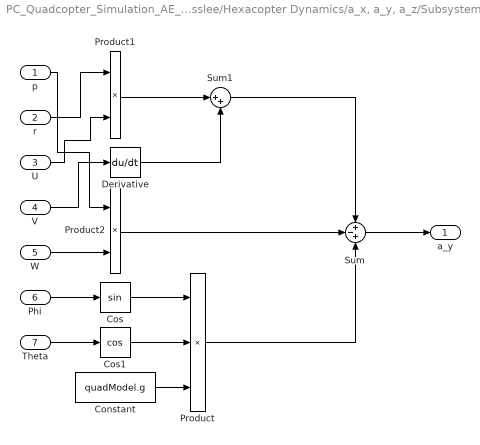
== system PC_Quadcopter_Simulation_AE_sslee/Hexacopter Dynamics/a_x, a_y, a_z/Subsystem1 ==
  p : Inport
  r : Inport  Port=2
  U : Inport  Port=3
  V : Inport  Port=4
  W : Inport  Port=5
  Phi : Inport  Port=6
  Theta : Inport  Port=7
  Constant : Constant  Value=quadModel.g
  Cos : Trigonometry
  Cos1 : Trigonometry  Operator=cos
  Derivative : Derivative
  Product : Product  Inputs=3
  Product1 : Product
  Product2 : Product
  Sum : Sum  Inputs=+-+
  Sum1 : Sum  Inputs=|++
  a_y : Outport
  wires:
  V/1 -> Derivative/1
  Theta/1 -> Cos1/1
  Phi/1 -> Cos/1
  Cos/1 -> Product/1
  Cos1/1 -> Product/2
  Constant/1 -> Product/3
  Derivative/1 -> Sum1/2
  r/1 -> Product1/1
  U/1 -> Product1/2
  W/1 -> Product2/2
  p/1 -> Product2/1
  Product1/1 -> Sum1/1
  Product2/1 -> Sum/2
  Sum1/1 -> Sum/1
  Product/1 -> Sum/3
  Sum/1 -> a_y/1

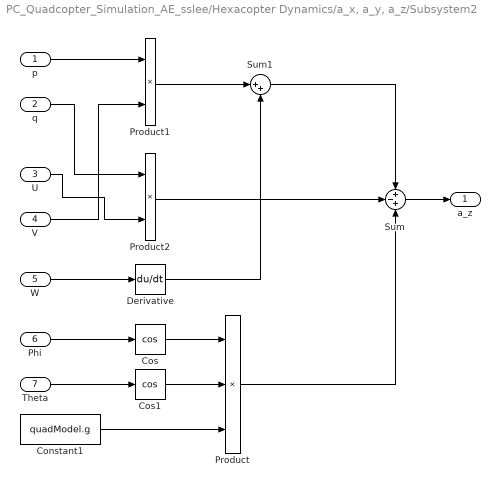
== system PC_Quadcopter_Simulation_AE_sslee/Hexacopter Dynamics/a_x, a_y, a_z/Subsystem2 ==
  p : Inport
  q : Inport  Port=2
  U : Inport  Port=3
  V : Inport  Port=4
  W : Inport  Port=5
  Phi : Inport  Port=6
  Theta : Inport  Port=7
  Constant1 : Constant  Value=quadModel.g
  Cos : Trigonometry  Operator=cos
  Cos1 : Trigonometry  Operator=cos
  Derivative : Derivative
  Product : Product  Inputs=3
  Product1 : Product
  Product2 : Product
  Sum : Sum  Inputs=+-+
  Sum1 : Sum  Inputs=|++
  a_z : Outport
  wires:
  Cos1/1 -> Product/2
  Constant1/1 -> Product/3
  Cos/1 -> Product/1
  Sum/1 -> a_z/1
  Theta/1 -> Cos1/1
  Phi/1 -> Cos/1
  W/1 -> Derivative/1
  p/1 -> Product1/1
  V/1 -> Product1/2
  q/1 -> Product2/1
  U/1 -> Product2/2
  Product1/1 -> Sum1/1
  Derivative/1 -> Sum1/2
  Product2/1 -> Sum/2
  Sum1/1 -> Sum/1
  Product/1 -> Sum/3

== matlab function PC_Quadcopter_Simulation_AE_sslee/Hexacopter Control Mixing/MATLAB Function ==
  data: u input; y output
function y = fcn(u)
%% mixing matrix: PID correction to motors
m = 1.023;
g = 9.81;
ct = 1.4865e-07;
cr = 80.5840;
b = 976.2;
%% health state 6*1
h = u(5:10,1);
FDI = u(11,1);
% 
% A = [
%     -1/h(1,1) -1/h(1,1) -1/h(1,1) 1/h(1,1)
%     1/h(2,1) -1/h(2,1) 1/h(2,1) 1/h(2,1)
%     1/h(3,1) 0 -1/h(3,1) 1/h(3,1)
%     1/h(4,1) 1/h(4,1) 1/h(4,1) 1/h(4,1)
%     -1/h(5,1) 1/h(5,1) -1/h(5,1) 1/h(5,1)
%     -1/h(6,1) 0 1/h(6,1) 1/h(6,1)
%     ];

A = [
    -1 -1 -1 1
    1 -1 1 1
    1 0 -1 1
    1 1 1 1
    -1 1 -1 1
    -1 0 1 1
    ];

%% 고장을 고려한 mixing 변화
if FDI==1 | FDI==4
h(1,1)=0;
h(2,1)=1;
h(3,1)=1;
h(4,1)=0;
h(5,1)=1;
h(6,1)=1;

A = [
    -1 -1 -1 1
    1 -1 1 1
    1 0 -1 1
    1 1 1 1
    -1 1 -1 1
    -1 0 1 1
    ];

elseif FDI==2 | FDI==5
h(1,1)=1;
h(2,1)=0;
h(3,1)=1;
h(4,1)=1;
h(5,1)=0;
h(6,1)=1;

A = [
    -1 -1 -1 1
    1 -1 1 1
    1 0 -1 1
    1 1 1 1
    -1 1 -1 1
    -1 0 1 1
    ];

elseif FDI==3 | FDI==6
h(1,1)=1;
h(2,1)=1;
h(3,1)=0;
h(4,1)=1;
h(5,1)=1;
h(6,1)=0;
% 
A = [
    -1 -1 -1 1
    1 -1 1 1
    1 0 -1 1
    1 1 1 1
    -1 1 -1 1
    -1 0 1 1
    ];

end
for i=1:6
    A(i,:) = h(i)*A(i,:);
end

%% 고장을 고려한 건강한 모터의 추력 증가
% A = sqrt(6/sum(h))*A;


y = A*( u(1:4,:) )
% y = A*( u(1:4,:) ) + (sqrt(m*g/sum(h)/ct)-b)/cr ...
%     - (sqrt(m*g/6/ct)-b)/cr ;
